simulink model "projectParallel"  (R2015b)
settings: Solver=FixedStepDiscrete  SolverMode=SingleTasking  StartTime=0.0  StopTime=10.0  RelTol=1e-3
libraries: shlslibv1 x202
settings Model: synDspstartup=OK  Creator=sdatta24  LastModifiedBy=agill17
settings DataIOCC: SaveOutput=off  SignalLogging=off  SaveTime=off
settings OptimizationCC: DefaultParameterBehavior=Inlined
settings DebuggingCC: AlgebraicLoopMsg=error  InheritedTsInSrcMsg=none

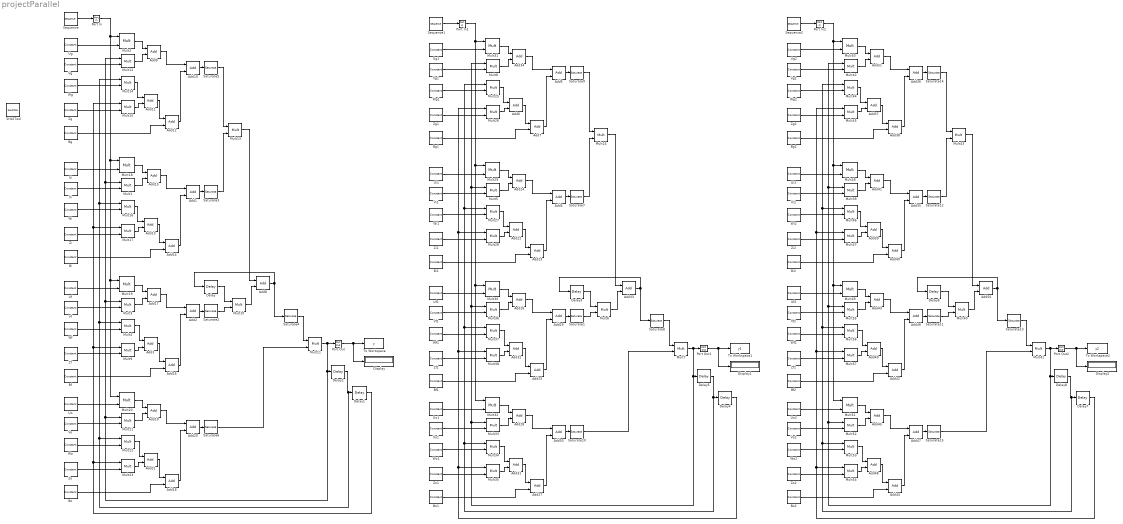
== system projectParallel ==
  Add{1..2,4..5,10,29,35..36,46} (9 alike) : shlslibv1/Math Functions/Add  syn_add_opr=++  syn_out_f=Full Precision  syn_out_wl=16  syn_out_fl=8  syn_out_dt=signed  syn_out_sat=off  syn_out_rnd=Floor (Truncate)  synBlockType=primitive  synLatency=0  synBlockId=96  syn_sum_of_rows=off  syn_inh_port=off  syn_inh_st=on  syn_inh_stf=1  syn_en_pipe=off  syn_pipe_stg=syn_max_pipeline  syn_flow_ctrl=off
  Add{3,6..8,11..14,16,18,21..23,25,27,31..33,37..40,42,44,48..50} (27 alike) : shlslibv1/Math Functions/Add  syn_add_opr=++  syn_out_f=Specify  syn_out_wl=25  syn_out_fl=7  syn_out_dt=unsigned  syn_out_sat=off  syn_out_rnd=Floor (Truncate)  synBlockType=primitive  synLatency=0  synBlockId=96  syn_sum_of_rows=off  syn_inh_port=off  syn_inh_st=on  syn_inh_stf=1  syn_en_pipe=off  syn_pipe_stg=syn_max_pipeline  syn_flow_ctrl=off
  Add{9,15,17,19,24,26,28,34,41,43,45,51} (12 alike) : shlslibv1/Math Functions/Add  syn_add_opr=++  syn_out_f=Specify  syn_out_wl=25  syn_out_fl=7  syn_out_dt=unsigned  syn_out_sat=off  syn_out_rnd=Floor (Truncate)  synBlockType=primitive  synLatency=0  synBlockId=96  syn_sum_of_rows=off  syn_inh_port=off  syn_inh_st=on  syn_inh_stf=1  syn_en_pipe=on  syn_pipe_stg=2  syn_flow_ctrl=off
  Add20 : shlslibv1/Math Functions/Add  syn_add_opr=++  syn_out_f=Full Precision  syn_out_wl=16  syn_out_fl=8  syn_out_dt=signed  syn_out_sat=off  syn_out_rnd=Floor (Truncate)  synBlockType=primitive  synLatency=0  synBlockId=96  syn_sum_of_rows=off  syn_inh_port=off  syn_inh_st=on  syn_inh_stf=1  syn_en_pipe=on  syn_pipe_stg=4  syn_flow_ctrl=off
  Add30 : shlslibv1/Math Functions/Add  syn_add_opr=++  syn_out_f=Full Precision  syn_out_wl=16  syn_out_fl=8  syn_out_dt=signed  syn_out_sat=off  syn_out_rnd=Floor (Truncate)  synBlockType=primitive  synLatency=0  synBlockId=96  syn_sum_of_rows=off  syn_inh_port=off  syn_inh_st=on  syn_inh_stf=1  syn_en_pipe=on  syn_pipe_stg=4  syn_flow_ctrl=off
  Add47 : shlslibv1/Math Functions/Add  syn_add_opr=++  syn_out_f=Full Precision  syn_out_wl=16  syn_out_fl=8  syn_out_dt=signed  syn_out_sat=off  syn_out_rnd=Floor (Truncate)  synBlockType=primitive  synLatency=0  synBlockId=96  syn_sum_of_rows=off  syn_inh_port=off  syn_inh_st=on  syn_inh_stf=1  syn_en_pipe=on  syn_pipe_stg=4  syn_flow_ctrl=off
  Bf : shlslibv1/Sources/Constant  syn_cst_val=1  syn_cst_format=Specify  syn_cst_wl=25  syn_cst_fl=7  syn_cst_dt=unsigned  syn_cst_rnd=on  syn_cst_st=1/300e6  synBlockType=primitive  synLatency=0  synBlockId=15
  Bf1 : shlslibv1/Sources/Constant  syn_cst_val=1  syn_cst_format=Specify  syn_cst_wl=25  syn_cst_fl=7  syn_cst_dt=unsigned  syn_cst_rnd=on  syn_cst_st=1/300e6  synBlockType=primitive  synLatency=0  synBlockId=15
  Bf2 : shlslibv1/Sources/Constant  syn_cst_val=1  syn_cst_format=Specify  syn_cst_wl=25  syn_cst_fl=7  syn_cst_dt=unsigned  syn_cst_rnd=on  syn_cst_st=1/300e6  synBlockType=primitive  synLatency=0  synBlockId=15
  Bg : shlslibv1/Sources/Constant  syn_cst_val=1  syn_cst_format=Specify  syn_cst_wl=25  syn_cst_fl=7  syn_cst_dt=unsigned  syn_cst_rnd=on  syn_cst_st=1/300e6  synBlockType=primitive  synLatency=0  synBlockId=15
  Bg1 : shlslibv1/Sources/Constant  syn_cst_val=1  syn_cst_format=Specify  syn_cst_wl=25  syn_cst_fl=7  syn_cst_dt=unsigned  syn_cst_rnd=on  syn_cst_st=1/300e6  synBlockType=primitive  synLatency=0  synBlockId=15
  Bg2 : shlslibv1/Sources/Constant  syn_cst_val=1  syn_cst_format=Specify  syn_cst_wl=25  syn_cst_fl=7  syn_cst_dt=unsigned  syn_cst_rnd=on  syn_cst_st=1/300e6  synBlockType=primitive  synLatency=0  synBlockId=15
  Bi : shlslibv1/Sources/Constant  syn_cst_val=1  syn_cst_format=Specify  syn_cst_wl=25  syn_cst_fl=7  syn_cst_dt=unsigned  syn_cst_rnd=on  syn_cst_st=1/300e6  synBlockType=primitive  synLatency=0  synBlockId=15
  Bi1 : shlslibv1/Sources/Constant  syn_cst_val=1  syn_cst_format=Specify  syn_cst_wl=25  syn_cst_fl=7  syn_cst_dt=unsigned  syn_cst_rnd=on  syn_cst_st=1/300e6  synBlockType=primitive  synLatency=0  synBlockId=15
  Bi2 : shlslibv1/Sources/Constant  syn_cst_val=1  syn_cst_format=Specify  syn_cst_wl=25  syn_cst_fl=7  syn_cst_dt=unsigned  syn_cst_rnd=on  syn_cst_st=1/300e6  synBlockType=primitive  synLatency=0  synBlockId=15
  Bo : shlslibv1/Sources/Constant  syn_cst_val=1  syn_cst_format=Specify  syn_cst_wl=25  syn_cst_fl=7  syn_cst_dt=unsigned  syn_cst_rnd=on  syn_cst_st=1/300e6  synBlockType=primitive  synLatency=0  synBlockId=15
  Bo1 : shlslibv1/Sources/Constant  syn_cst_val=1  syn_cst_format=Specify  syn_cst_wl=25  syn_cst_fl=7  syn_cst_dt=unsigned  syn_cst_rnd=on  syn_cst_st=1/300e6  synBlockType=primitive  synLatency=0  synBlockId=15
  Bo2 : shlslibv1/Sources/Constant  syn_cst_val=1  syn_cst_format=Specify  syn_cst_wl=25  syn_cst_fl=7  syn_cst_dt=unsigned  syn_cst_rnd=on  syn_cst_st=1/300e6  synBlockType=primitive  synLatency=0  synBlockId=15
  Delay : shlslibv1/Memories/Delay  syn_delay_val=1  synBlockType=primitive  synLatency=1  synBlockId=104
  Delay{1..2,4..5,7..8} (6 alike) : shlslibv1/Memories/Delay  syn_delay_val=9  synBlockType=primitive  synLatency=9  synBlockId=104
  Delay3 : shlslibv1/Memories/Delay  syn_delay_val=1  synBlockType=primitive  synLatency=1  synBlockId=104
  Delay6 : shlslibv1/Memories/Delay  syn_delay_val=1  synBlockType=primitive  synLatency=1  synBlockId=104
  Display : Display
  Display1 : Display
  Display2 : Display
  Mult{1..57} (57 alike) : shlslibv1/Math Functions/Mult  syn_out_f=Specify  syn_out_wl=25  syn_out_fl=7  syn_out_dt=unsigned  syn_out_sat=off  syn_out_rnd=Floor (Truncate)  syn_inh_port=off  syn_inh_st=off  syn_inh_stf=1  syn_en_pipe=off  syn_pipe_stg=syn_max_pipeline  syn_flow_ctrl=off  synBlockType=primitive  synLatency=0  synBlockId=3  syn_opr_mode=1
  Port In : shlslibv1/Ports & Subsystems/Port In  syn_out_wl=25  syn_out_fl=7  syn_out_dt=unsigned  syn_out_st=1/300e6  syn_capture=on  syn_register=on  syn_out_sat=off  syn_out_rnd=on  synBlockType=port  synLatency=1  synBlockId=0
  Port In1 : shlslibv1/Ports & Subsystems/Port In  syn_out_wl=25  syn_out_fl=7  syn_out_dt=unsigned  syn_out_st=1/300e6  syn_capture=on  syn_register=on  syn_out_sat=off  syn_out_rnd=on  synBlockType=port  synLatency=1  synBlockId=0
  Port In2 : shlslibv1/Ports & Subsystems/Port In  syn_out_wl=25  syn_out_fl=7  syn_out_dt=unsigned  syn_out_st=1/300e6  syn_capture=on  syn_register=on  syn_out_sat=off  syn_out_rnd=on  synBlockType=port  synLatency=1  synBlockId=0
  Port Out : shlslibv1/Ports & Subsystems/Port Out  syn_capture=on  syn_register=on  synBlockType=port  synLatency=1  synBlockId=1
  Port Out1 : shlslibv1/Ports & Subsystems/Port Out  syn_capture=on  syn_register=on  synBlockType=port  synLatency=1  synBlockId=1
  Port Out2 : shlslibv1/Ports & Subsystems/Port Out  syn_capture=on  syn_register=on  synBlockType=port  synLatency=1  synBlockId=1
  SHLSTool : shlslibv1/SHLSTool  synBlockType=tool  syn_dsp_mode=FPGA
  Saturate{1..3,6..7,10..12,15} (9 alike) : shlslibv1/Signal Operations/Saturate  syn_sat_mode=Constant  syn_pos_val=1  syn_neg_val=0  syn_sat_fl=7  syn_sat_rnd=on  syn_out_f=Same as Input  syn_out_wl=16  syn_out_fl=15  syn_out_dt=signed  syn_out_rnd=on  syn_pipe=on  syn_sat_ind=off  synBlockType=custom  synLatency=1
  Saturate{4..5,8..9,13..14} (6 alike) : shlslibv1/Signal Operations/Saturate  syn_sat_mode=Constant  syn_pos_val=1  syn_neg_val=-1  syn_sat_fl=7  syn_sat_rnd=on  syn_out_f=Same as Input  syn_out_wl=16  syn_out_fl=15  syn_out_dt=signed  syn_out_rnd=on  syn_pipe=on  syn_sat_ind=off  synBlockType=custom  synLatency=1
  Sequence : shlslibv1/Sources/Sequence  syn_seq_vec=[100 100 100 100 100 100 100 100 100 200 200 200 200 200 200 200 200 200 300 300 300 300 300 300 300 300 300 400 400 400 400 400 400 400 400 400 500 500 500 500 500 500 500 500 500 600 600 600 600 600 600 600 600 600 700 700 700 700 700 700 700 700 700 800 800 800 800 800 800 800 800 800 900 900 900 900 900 900 900 900 900]  syn_seq_wl=25  syn_seq_fl=7  syn_seq_dt=unsigned  syn_rst_port=off  syn_en_port=off  syn_seq_st=1/300e6  synBlockType=custom  synLatency=1
  Sequence1 : shlslibv1/Sources/Sequence  syn_seq_vec=[100 100 100 100 100 100 100 100 100 200 200 200 200 200 200 200 200 200 300 300 300 300 300 300 300 300 300 400 400 400 400 400 400 400 400 400 500 500 500 500 500 500 500 500 500 600 600 600 600 600 600 600 600 600 700 700 700 700 700 700 700 700 700 800 800 800 800 800 800 800 800 800 900 900 900 900 900 900 900 900 900]  syn_seq_wl=25  syn_seq_fl=7  syn_seq_dt=unsigned  syn_rst_port=off  syn_en_port=off  syn_seq_st=1/300e6  synBlockType=custom  synLatency=1
  Sequence2 : shlslibv1/Sources/Sequence  syn_seq_vec=[100 100 100 100 100 100 100 100 100 200 200 200 200 200 200 200 200 200 300 300 300 300 300 300 300 300 300 400 400 400 400 400 400 400 400 400 500 500 500 500 500 500 500 500 500 600 600 600 600 600 600 600 600 600 700 700 700 700 700 700 700 700 700 800 800 800 800 800 800 800 800 800 900 900 900 900 900 900 900 900 900]  syn_seq_wl=25  syn_seq_fl=7  syn_seq_dt=unsigned  syn_rst_port=off  syn_en_port=off  syn_seq_st=1/300e6  synBlockType=custom  synLatency=1
  To Workspace : ToWorkspace  VariableName=y  SaveFormat=Structure With Time  SampleTime=1/320e6
  To Workspace1 : ToWorkspace  VariableName=y1  SaveFormat=Structure With Time  SampleTime=1/320e6
  To Workspace2 : ToWorkspace  VariableName=y2  SaveFormat=Structure With Time  SampleTime=1/320e6
  Uf : shlslibv1/Sources/Constant  syn_cst_val=0  syn_cst_format=Specify  syn_cst_wl=25  syn_cst_fl=7  syn_cst_dt=unsigned  syn_cst_rnd=on  syn_cst_st=1/300e6  synBlockType=primitive  synLatency=0  synBlockId=15
  Uf1 : shlslibv1/Sources/Constant  syn_cst_val=0  syn_cst_format=Specify  syn_cst_wl=25  syn_cst_fl=7  syn_cst_dt=unsigned  syn_cst_rnd=on  syn_cst_st=1/300e6  synBlockType=primitive  synLatency=0  synBlockId=15
  Uf2 : shlslibv1/Sources/Constant  syn_cst_val=0  syn_cst_format=Specify  syn_cst_wl=25  syn_cst_fl=7  syn_cst_dt=unsigned  syn_cst_rnd=on  syn_cst_st=1/300e6  synBlockType=primitive  synLatency=0  synBlockId=15
  Ug : shlslibv1/Sources/Constant  syn_cst_val=1  syn_cst_format=Specify  syn_cst_wl=25  syn_cst_fl=7  syn_cst_dt=unsigned  syn_cst_rnd=on  syn_cst_st=1/300e6  synBlockType=primitive  synLatency=0  synBlockId=15
  Ug1 : shlslibv1/Sources/Constant  syn_cst_val=1  syn_cst_format=Specify  syn_cst_wl=25  syn_cst_fl=7  syn_cst_dt=unsigned  syn_cst_rnd=on  syn_cst_st=1/300e6  synBlockType=primitive  synLatency=0  synBlockId=15
  Ug2 : shlslibv1/Sources/Constant  syn_cst_val=1  syn_cst_format=Specify  syn_cst_wl=25  syn_cst_fl=7  syn_cst_dt=unsigned  syn_cst_rnd=on  syn_cst_st=1/300e6  synBlockType=primitive  synLatency=0  synBlockId=15
  Ui : shlslibv1/Sources/Constant  syn_cst_val=1  syn_cst_format=Specify  syn_cst_wl=25  syn_cst_fl=7  syn_cst_dt=unsigned  syn_cst_rnd=on  syn_cst_st=1/300e6  synBlockType=primitive  synLatency=0  synBlockId=15
  Ui1 : shlslibv1/Sources/Constant  syn_cst_val=1  syn_cst_format=Specify  syn_cst_wl=25  syn_cst_fl=7  syn_cst_dt=unsigned  syn_cst_rnd=on  syn_cst_st=1/300e6  synBlockType=primitive  synLatency=0  synBlockId=15
  Ui2 : shlslibv1/Sources/Constant  syn_cst_val=1  syn_cst_format=Specify  syn_cst_wl=25  syn_cst_fl=7  syn_cst_dt=unsigned  syn_cst_rnd=on  syn_cst_st=1/300e6  synBlockType=primitive  synLatency=0  synBlockId=15
  Uo : shlslibv1/Sources/Constant  syn_cst_val=1  syn_cst_format=Specify  syn_cst_wl=25  syn_cst_fl=7  syn_cst_dt=unsigned  syn_cst_rnd=on  syn_cst_st=1/300e6  synBlockType=primitive  synLatency=0  synBlockId=15
  Uo1 : shlslibv1/Sources/Constant  syn_cst_val=1  syn_cst_format=Specify  syn_cst_wl=25  syn_cst_fl=7  syn_cst_dt=unsigned  syn_cst_rnd=on  syn_cst_st=1/300e6  synBlockType=primitive  synLatency=0  synBlockId=15
  Uo2 : shlslibv1/Sources/Constant  syn_cst_val=1  syn_cst_format=Specify  syn_cst_wl=25  syn_cst_fl=7  syn_cst_dt=unsigned  syn_cst_rnd=on  syn_cst_st=1/300e6  synBlockType=primitive  synLatency=0  synBlockId=15
  Vf : shlslibv1/Sources/Constant  syn_cst_val=0  syn_cst_format=Specify  syn_cst_wl=25  syn_cst_fl=7  syn_cst_dt=unsigned  syn_cst_rnd=on  syn_cst_st=1/300e6  synBlockType=primitive  synLatency=0  synBlockId=15
  Vf1 : shlslibv1/Sources/Constant  syn_cst_val=0  syn_cst_format=Specify  syn_cst_wl=25  syn_cst_fl=7  syn_cst_dt=unsigned  syn_cst_rnd=on  syn_cst_st=1/300e6  synBlockType=primitive  synLatency=0  synBlockId=15
  Vf2 : shlslibv1/Sources/Constant  syn_cst_val=0  syn_cst_format=Specify  syn_cst_wl=25  syn_cst_fl=7  syn_cst_dt=unsigned  syn_cst_rnd=on  syn_cst_st=1/300e6  synBlockType=primitive  synLatency=0  synBlockId=15
  Vg : shlslibv1/Sources/Constant  syn_cst_val=1  syn_cst_format=Specify  syn_cst_wl=25  syn_cst_fl=7  syn_cst_dt=unsigned  syn_cst_rnd=on  syn_cst_st=1/300e6  synBlockType=primitive  synLatency=0  synBlockId=15
  Vg1 : shlslibv1/Sources/Constant  syn_cst_val=1  syn_cst_format=Specify  syn_cst_wl=25  syn_cst_fl=7  syn_cst_dt=unsigned  syn_cst_rnd=on  syn_cst_st=1/300e6  synBlockType=primitive  synLatency=0  synBlockId=15
  Vg2 : shlslibv1/Sources/Constant  syn_cst_val=1  syn_cst_format=Specify  syn_cst_wl=25  syn_cst_fl=7  syn_cst_dt=unsigned  syn_cst_rnd=on  syn_cst_st=1/300e6  synBlockType=primitive  synLatency=0  synBlockId=15
  Vi : shlslibv1/Sources/Constant  syn_cst_val=1  syn_cst_format=Specify  syn_cst_wl=25  syn_cst_fl=7  syn_cst_dt=unsigned  syn_cst_rnd=on  syn_cst_st=1/300e6  synBlockType=primitive  synLatency=0  synBlockId=15
  Vi1 : shlslibv1/Sources/Constant  syn_cst_val=1  syn_cst_format=Specify  syn_cst_wl=25  syn_cst_fl=7  syn_cst_dt=unsigned  syn_cst_rnd=on  syn_cst_st=1/300e6  synBlockType=primitive  synLatency=0  synBlockId=15
  Vi2 : shlslibv1/Sources/Constant  syn_cst_val=1  syn_cst_format=Specify  syn_cst_wl=25  syn_cst_fl=7  syn_cst_dt=unsigned  syn_cst_rnd=on  syn_cst_st=1/300e6  synBlockType=primitive  synLatency=0  synBlockId=15
  Vo : shlslibv1/Sources/Constant  syn_cst_val=1  syn_cst_format=Specify  syn_cst_wl=25  syn_cst_fl=7  syn_cst_dt=unsigned  syn_cst_rnd=on  syn_cst_st=1/300e6  synBlockType=primitive  synLatency=0  synBlockId=15
  Vo1 : shlslibv1/Sources/Constant  syn_cst_val=1  syn_cst_format=Specify  syn_cst_wl=25  syn_cst_fl=7  syn_cst_dt=unsigned  syn_cst_rnd=on  syn_cst_st=1/300e6  synBlockType=primitive  synLatency=0  synBlockId=15
  Vo2 : shlslibv1/Sources/Constant  syn_cst_val=1  syn_cst_format=Specify  syn_cst_wl=25  syn_cst_fl=7  syn_cst_dt=unsigned  syn_cst_rnd=on  syn_cst_st=1/300e6  synBlockType=primitive  synLatency=0  synBlockId=15
  Wf : shlslibv1/Sources/Constant  syn_cst_val=0  syn_cst_format=Specify  syn_cst_wl=25  syn_cst_fl=7  syn_cst_dt=unsigned  syn_cst_rnd=on  syn_cst_st=1/300e6  synBlockType=primitive  synLatency=0  synBlockId=15
  Wf1 : shlslibv1/Sources/Constant  syn_cst_val=0  syn_cst_format=Specify  syn_cst_wl=25  syn_cst_fl=7  syn_cst_dt=unsigned  syn_cst_rnd=on  syn_cst_st=1/300e6  synBlockType=primitive  synLatency=0  synBlockId=15
  Wf2 : shlslibv1/Sources/Constant  syn_cst_val=0  syn_cst_format=Specify  syn_cst_wl=25  syn_cst_fl=7  syn_cst_dt=unsigned  syn_cst_rnd=on  syn_cst_st=1/300e6  synBlockType=primitive  synLatency=0  synBlockId=15
  Wg : shlslibv1/Sources/Constant  syn_cst_val=1  syn_cst_format=Specify  syn_cst_wl=25  syn_cst_fl=7  syn_cst_dt=unsigned  syn_cst_rnd=on  syn_cst_st=1/300e6  synBlockType=primitive  synLatency=0  synBlockId=15
  Wg1 : shlslibv1/Sources/Constant  syn_cst_val=1  syn_cst_format=Specify  syn_cst_wl=25  syn_cst_fl=7  syn_cst_dt=unsigned  syn_cst_rnd=on  syn_cst_st=1/300e6  synBlockType=primitive  synLatency=0  synBlockId=15
  Wg2 : shlslibv1/Sources/Constant  syn_cst_val=1  syn_cst_format=Specify  syn_cst_wl=25  syn_cst_fl=7  syn_cst_dt=unsigned  syn_cst_rnd=on  syn_cst_st=1/300e6  synBlockType=primitive  synLatency=0  synBlockId=15
  Wi : shlslibv1/Sources/Constant  syn_cst_val=1  syn_cst_format=Specify  syn_cst_wl=25  syn_cst_fl=7  syn_cst_dt=unsigned  syn_cst_rnd=on  syn_cst_st=1/300e6  synBlockType=primitive  synLatency=0  synBlockId=15
  Wi1 : shlslibv1/Sources/Constant  syn_cst_val=1  syn_cst_format=Specify  syn_cst_wl=25  syn_cst_fl=7  syn_cst_dt=unsigned  syn_cst_rnd=on  syn_cst_st=1/300e6  synBlockType=primitive  synLatency=0  synBlockId=15
  Wi2 : shlslibv1/Sources/Constant  syn_cst_val=1  syn_cst_format=Specify  syn_cst_wl=25  syn_cst_fl=7  syn_cst_dt=unsigned  syn_cst_rnd=on  syn_cst_st=1/300e6  synBlockType=primitive  synLatency=0  synBlockId=15
  Wo : shlslibv1/Sources/Constant  syn_cst_val=1  syn_cst_format=Specify  syn_cst_wl=25  syn_cst_fl=7  syn_cst_dt=unsigned  syn_cst_rnd=on  syn_cst_st=1/300e6  synBlockType=primitive  synLatency=0  synBlockId=15
  Wo1 : shlslibv1/Sources/Constant  syn_cst_val=1  syn_cst_format=Specify  syn_cst_wl=25  syn_cst_fl=7  syn_cst_dt=unsigned  syn_cst_rnd=on  syn_cst_st=1/300e6  synBlockType=primitive  synLatency=0  synBlockId=15
  Wo2 : shlslibv1/Sources/Constant  syn_cst_val=1  syn_cst_format=Specify  syn_cst_wl=25  syn_cst_fl=7  syn_cst_dt=unsigned  syn_cst_rnd=on  syn_cst_st=1/300e6  synBlockType=primitive  synLatency=0  synBlockId=15
  Zf : shlslibv1/Sources/Constant  syn_cst_val=0  syn_cst_format=Specify  syn_cst_wl=25  syn_cst_fl=7  syn_cst_dt=unsigned  syn_cst_rnd=on  syn_cst_st=1/300e6  synBlockType=primitive  synLatency=0  synBlockId=15
  Zf1 : shlslibv1/Sources/Constant  syn_cst_val=0  syn_cst_format=Specify  syn_cst_wl=25  syn_cst_fl=7  syn_cst_dt=unsigned  syn_cst_rnd=on  syn_cst_st=1/300e6  synBlockType=primitive  synLatency=0  synBlockId=15
  Zf2 : shlslibv1/Sources/Constant  syn_cst_val=0  syn_cst_format=Specify  syn_cst_wl=25  syn_cst_fl=7  syn_cst_dt=unsigned  syn_cst_rnd=on  syn_cst_st=1/300e6  synBlockType=primitive  synLatency=0  synBlockId=15
  Zg : shlslibv1/Sources/Constant  syn_cst_val=1  syn_cst_format=Specify  syn_cst_wl=25  syn_cst_fl=7  syn_cst_dt=unsigned  syn_cst_rnd=on  syn_cst_st=1/300e6  synBlockType=primitive  synLatency=0  synBlockId=15
  Zg1 : shlslibv1/Sources/Constant  syn_cst_val=1  syn_cst_format=Specify  syn_cst_wl=25  syn_cst_fl=7  syn_cst_dt=unsigned  syn_cst_rnd=on  syn_cst_st=1/300e6  synBlockType=primitive  synLatency=0  synBlockId=15
  Zg2 : shlslibv1/Sources/Constant  syn_cst_val=1  syn_cst_format=Specify  syn_cst_wl=25  syn_cst_fl=7  syn_cst_dt=unsigned  syn_cst_rnd=on  syn_cst_st=1/300e6  synBlockType=primitive  synLatency=0  synBlockId=15
  Zi : shlslibv1/Sources/Constant  syn_cst_val=1  syn_cst_format=Specify  syn_cst_wl=25  syn_cst_fl=7  syn_cst_dt=unsigned  syn_cst_rnd=on  syn_cst_st=1/300e6  synBlockType=primitive  synLatency=0  synBlockId=15
  Zi1 : shlslibv1/Sources/Constant  syn_cst_val=1  syn_cst_format=Specify  syn_cst_wl=25  syn_cst_fl=7  syn_cst_dt=unsigned  syn_cst_rnd=on  syn_cst_st=1/300e6  synBlockType=primitive  synLatency=0  synBlockId=15
  Zi2 : shlslibv1/Sources/Constant  syn_cst_val=1  syn_cst_format=Specify  syn_cst_wl=25  syn_cst_fl=7  syn_cst_dt=unsigned  syn_cst_rnd=on  syn_cst_st=1/300e6  synBlockType=primitive  synLatency=0  synBlockId=15
  Zo : shlslibv1/Sources/Constant  syn_cst_val=1  syn_cst_format=Specify  syn_cst_wl=25  syn_cst_fl=7  syn_cst_dt=unsigned  syn_cst_rnd=on  syn_cst_st=1/300e6  synBlockType=primitive  synLatency=0  synBlockId=15
  Zo1 : shlslibv1/Sources/Constant  syn_cst_val=1  syn_cst_format=Specify  syn_cst_wl=25  syn_cst_fl=7  syn_cst_dt=unsigned  syn_cst_rnd=on  syn_cst_st=1/300e6  synBlockType=primitive  synLatency=0  synBlockId=15
  Zo2 : shlslibv1/Sources/Constant  syn_cst_val=1  syn_cst_format=Specify  syn_cst_wl=25  syn_cst_fl=7  syn_cst_dt=unsigned  syn_cst_rnd=on  syn_cst_st=1/300e6  synBlockType=primitive  synLatency=0  synBlockId=15
  wires:
  Sequence/1 -> Port In/1
  Ug/1 -> Mult2/2
  Vg/1 -> Mult12/2
  Mult2/1 -> Add9/1
  Mult12/1 -> Add9/2
  Add9/1 -> Add10/1
  Add10/1 -> Saturate5/1
  Saturate5/1 -> Mult13/1
  Wg/1 -> Mult14/2
  Zg/1 -> Mult15/2
  Mult14/1 -> Add11/1
  Mult15/1 -> Add11/2
  Add11/1 -> Add12/1
  Bg/1 -> Add12/2
  Add12/1 -> Add10/2
  Ui/1 -> Mult18/2
  Vi/1 -> Mult1/2
  Mult18/1 -> Add15/1
  Mult1/1 -> Add15/2
  Add15/1 -> Add1/1
  Add1/1 -> Saturate3/1
  Wi/1 -> Mult16/2
  Zi/1 -> Mult17/2
  Mult16/1 -> Add13/1
  Mult17/1 -> Add13/2
  Add13/1 -> Add14/1
  Bi/1 -> Add14/2
  Add14/1 -> Add1/2
  Saturate3/1 -> Mult13/2
  Uf/1 -> Mult19/2
  Vf/1 -> Mult3/2
  Mult19/1 -> Add17/1
  Mult3/1 -> Add17/2
  Add17/1 -> Add2/1
  Add2/1 -> Saturate2/1
  Wf/1 -> Mult4/2
  Zf/1 -> Mult9/2
  Mult4/1 -> Add3/1
  Mult9/1 -> Add3/2
  Add3/1 -> Add16/1
  Bf/1 -> Add16/2
  Add16/1 -> Add2/2
  Uo/1 -> Mult20/2
  Vo/1 -> Mult21/2
  Mult20/1 -> Add19/1
  Mult21/1 -> Add19/2
  Add19/1 -> Add20/1
  Add20/1 -> Saturate6/1
  Wo/1 -> Mult22/2
  Zo/1 -> Mult23/2
  Mult22/1 -> Add21/1
  Mult23/1 -> Add21/2
  Add21/1 -> Add18/1
  Bo/1 -> Add18/2
  Add18/1 -> Add20/2
  Mult11/1 -> Mult21/1, Mult3/1, Mult1/1, Mult12/1, Delay2/1, Port Out/1
  Delay/1 -> Mult10/1
  Mult10/1 -> Add8/2
  Add8/1 -> Delay/1, Saturate4/1
  Port Out/1 -> Display/1, To Workspace/1
  Saturate4/1 -> Mult11/1
  Saturate2/1 -> Mult10/2
  Mult13/1 -> Add8/1
  Saturate6/1 -> Mult11/2
  Delay2/1 -> Mult22/1, Mult4/1, Mult16/1, Mult14/1, Delay1/1
  Delay1/1 -> Mult23/1, Mult9/1, Mult17/1, Mult15/1
  Port In/1 -> Mult19/1, Mult20/1, Mult18/1, Mult2/1
  Sequence1/1 -> Port In1/1
  Ug1/1 -> Mult31/2
  Vg1/1 -> Mult8/2
  Mult31/1 -> Add34/1
  Mult8/1 -> Add34/2
  Add34/1 -> Add5/1
  Add5/1 -> Saturate9/1
  Saturate9/1 -> Mult24/1
  Wg1/1 -> Mult25/2
  Zg1/1 -> Mult26/2
  Mult25/1 -> Add6/1
  Mult26/1 -> Add6/2
  Add6/1 -> Add7/1
  Bg1/1 -> Add7/2
  Add7/1 -> Add5/2
  Ui1/1 -> Mult29/2
  Vi1/1 -> Mult5/2
  Mult29/1 -> Add24/1
  Mult5/1 -> Add24/2
  Add24/1 -> Add4/1
  Add4/1 -> Saturate7/1
  Wi1/1 -> Mult27/2
  Zi1/1 -> Mult28/2
  Mult27/1 -> Add22/1
  Mult28/1 -> Add22/2
  Add22/1 -> Add23/1
  Bi1/1 -> Add23/2
  Add23/1 -> Add4/2
  Saturate7/1 -> Mult24/2
  Uf1/1 -> Mult30/2
  Vf1/1 -> Mult36/2
  Mult30/1 -> Add26/1
  Mult36/1 -> Add26/2
  Add26/1 -> Add29/1
  Add29/1 -> Saturate1/1
  Wf1/1 -> Mult37/2
  Zf1/1 -> Mult38/2
  Mult37/1 -> Add32/1
  Mult38/1 -> Add32/2
  Add32/1 -> Add25/1
  Bf1/1 -> Add25/2
  Add25/1 -> Add29/2
  Uo1/1 -> Mult32/2
  Vo1/1 -> Mult33/2
  Mult32/1 -> Add28/1
  Mult33/1 -> Add28/2
  Add28/1 -> Add30/1
  Add30/1 -> Saturate10/1
  Wo1/1 -> Mult34/2
  Zo1/1 -> Mult35/2
  Mult34/1 -> Add31/1
  Mult35/1 -> Add31/2
  Add31/1 -> Add27/1
  Bo1/1 -> Add27/2
  Add27/1 -> Add30/2
  Mult7/1 -> Mult33/1, Mult36/1, Mult5/1, Mult8/1, Delay5/1, Port Out1/1
  Delay3/1 -> Mult6/1
  Mult6/1 -> Add33/2
  Add33/1 -> Delay3/1, Saturate8/1
  Port Out1/1 -> Display1/1, To Workspace1/1
  Saturate8/1 -> Mult7/1
  Saturate1/1 -> Mult6/2
  Mult24/1 -> Add33/1
  Saturate10/1 -> Mult7/2
  Delay5/1 -> Mult34/1, Mult37/1, Mult27/1, Mult25/1, Delay4/1
  Delay4/1 -> Mult35/1, Mult38/1, Mult28/1, Mult26/1
  Port In1/1 -> Mult30/1, Mult32/1, Mult29/1, Mult31/1
  Sequence2/1 -> Port In2/1
  Ug2/1 -> Mult50/2
  Vg2/1 -> Mult42/2
  Mult50/1 -> Add51/1
  Mult42/1 -> Add51/2
  Add51/1 -> Add36/1
  Add36/1 -> Saturate14/1
  Saturate14/1 -> Mult43/1
  Wg2/1 -> Mult44/2
  Zg2/1 -> Mult45/2
  Mult44/1 -> Add37/1
  Mult45/1 -> Add37/2
  Add37/1 -> Add38/1
  Bg2/1 -> Add38/2
  Add38/1 -> Add36/2
  Ui2/1 -> Mult48/2
  Vi2/1 -> Mult39/2
  Mult48/1 -> Add41/1
  Mult39/1 -> Add41/2
  Add41/1 -> Add35/1
  Add35/1 -> Saturate12/1
  Wi2/1 -> Mult46/2
  Zi2/1 -> Mult47/2
  Mult46/1 -> Add39/1
  Mult47/1 -> Add39/2
  Add39/1 -> Add40/1
  Bi2/1 -> Add40/2
  Add40/1 -> Add35/2
  Saturate12/1 -> Mult43/2
  Uf2/1 -> Mult49/2
  Vf2/1 -> Mult55/2
  Mult49/1 -> Add43/1
  Mult55/1 -> Add43/2
  Add43/1 -> Add46/1
  Add46/1 -> Saturate11/1
  Wf2/1 -> Mult56/2
  Zf2/1 -> Mult57/2
  Mult56/1 -> Add49/1
  Mult57/1 -> Add49/2
  Add49/1 -> Add42/1
  Bf2/1 -> Add42/2
  Add42/1 -> Add46/2
  Uo2/1 -> Mult51/2
  Vo2/1 -> Mult52/2
  Mult51/1 -> Add45/1
  Mult52/1 -> Add45/2
  Add45/1 -> Add47/1
  Add47/1 -> Saturate15/1
  Wo2/1 -> Mult53/2
  Zo2/1 -> Mult54/2
  Mult53/1 -> Add48/1
  Mult54/1 -> Add48/2
  Add48/1 -> Add44/1
  Bo2/1 -> Add44/2
  Add44/1 -> Add47/2
  Mult41/1 -> Mult52/1, Mult55/1, Mult39/1, Mult42/1, Delay8/1, Port Out2/1
  Delay6/1 -> Mult40/1
  Mult40/1 -> Add50/2
  Add50/1 -> Delay6/1, Saturate13/1
  Port Out2/1 -> Display2/1, To Workspace2/1
  Saturate13/1 -> Mult41/1
  Saturate11/1 -> Mult40/2
  Mult43/1 -> Add50/1
  Saturate15/1 -> Mult41/2
  Delay8/1 -> Mult53/1, Mult56/1, Mult46/1, Mult44/1, Delay7/1
  Delay7/1 -> Mult54/1, Mult57/1, Mult47/1, Mult45/1
  Port In2/1 -> Mult49/1, Mult51/1, Mult48/1, Mult50/1
